simulink model "Fuel_Fault_Detection"  (R2023b)
settings: Solver=FixedStepDiscrete  StartTime=0.0  StopTime=10.0  FixedStep=0.01  RelTol=1e-3
undefined symbols (not defined in the file): sigbuilder_block
libraries: simulink x5, Median_Filter_5th_lib x2, dspsrcs4 x1
settings Model: Creator=FAbdelkarim  LastModifiedBy=Farah
settings ModelReferenceCC: EnableRefExpFcnMdlSchedulingChecks=on

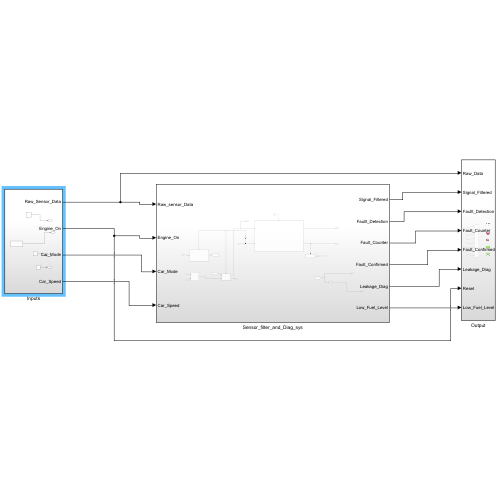
[thumbnail: Simulink's stored preview of the top-level diagram]
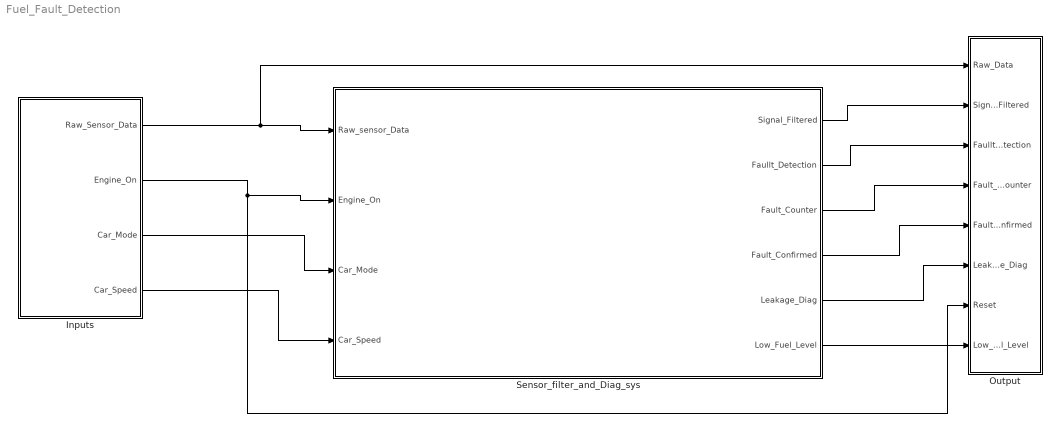
== system Fuel_Fault_Detection ==
  Inputs : Subsystem
  Output : Subsystem
  Sensor_filter_and_Diag_sys : Subsystem
  wires:
  Inputs/1(Raw_Sensor_Data) -> Output/1(Raw_Data), Sensor_filter_and_Diag_sys/1(Raw_sensor_Data)
  Inputs/2(Engine_On) -> Output/7(Reset), Sensor_filter_and_Diag_sys/2(Engine_On)
  Sensor_filter_and_Diag_sys/2(Faullt_Detection) -> Output/3(Faullt_Detection)
  Sensor_filter_and_Diag_sys/3(Fault_Counter) -> Output/4(Fault_Counter)
  Sensor_filter_and_Diag_sys/4(Fault_Confirmed) -> Output/5(Fault_Confirmed)
  Sensor_filter_and_Diag_sys/1(Signal_Filtered) -> Output/2(Signal_Filtered)
  Sensor_filter_and_Diag_sys/5(Leakage_Diag) -> Output/6(Leakage_Diag)
  Inputs/3(Car_Mode) -> Sensor_filter_and_Diag_sys/3(Car_Mode)
  Inputs/4(Car_Speed) -> Sensor_filter_and_Diag_sys/4(Car_Speed)
  Sensor_filter_and_Diag_sys/6(Low_Fuel_Level) -> Output/8(Low_Fuel_Level)

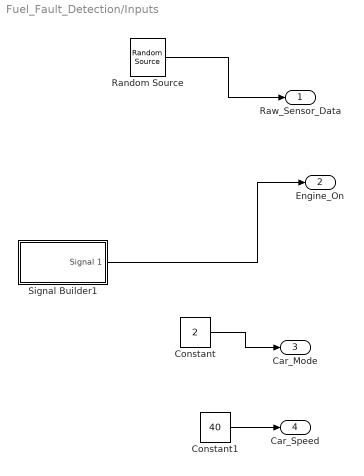
== system Fuel_Fault_Detection/Inputs ==
  Constant : Constant  Value=2
  Constant1 : Constant  Value=40
  Random Source : dspsrcs4/Random Source  SrcType=Uniform  NormMethod=Ziggurat  CltLength=12  MinVal=10  MaxVal=30  MeanVal=0  VarVal=1  RepMode=Not repeatable  rawSeed=1  IsInherit=off  SampMode=Discrete  SampTime=0.02  SampFrame=1  DataType=Double  OutComplex=Real  OutputFrames=off
  Signal Builder1 : Subsystem  Tag=STV Subsys  LoadFcn=sigbuilder_block('load');  StartFcn=sigbuilder_block('start');  StopFcn=sigbuilder_block('stop');  ClipboardFcn=sigbuilder_block('clipboard');  mask(Sigbuilder block){tuvar=[0:10]}
      mask help: Simulink:masks:SigbuilderBlock_MD
      mask init:
      | if ~strcmp(get_param(bdroot(gcbh),'SimulationStatus'),'stopped') tuvar = sigbuilder_block('maskInit'); end
      settings: CopyFcn=sigbuilder_block('copy');  DeleteFcn=sigbuilder_block('delete');  ModelCloseFcn=sigbuilder_block('modelClose');  PreSaveFcn=sigbuilder_block('preSave');  PauseFcn=sigbuilder_block('pause');  ContinueFcn=sigbuilder_block('continue');  NameChangeFcn=sigbuilder_block('namechange');  OpenFcn=sigbuilder_block('open',[437.6 199.2 550.4 400 ]);  CloseFcn=sigbuilder_block('close');
      mask Display: plot(0, 0, 100, 100,[2, 2, 32, 32, 2], [68, 8, 8, 68, 68],[32, 2], [38, 38], [32, 19, 2],[53, 60, 44], [32, 17, 17, 2],[16, 16, 31, 31]);txt = getActiveGroup(gcbh);text(2, 100, txt,'verticalAlignment', 'top');
  Raw_Sensor_Data : Outport
  Engine_On : Outport  Port=2
  Car_Mode : Outport  Port=3
  Car_Speed : Outport  Port=4
  wires:
  Random Source/1 -> Raw_Sensor_Data/1
  Signal Builder1/1(Signal 1) -> Engine_On/1
  Constant/1 -> Car_Mode/1
  Constant1/1 -> Car_Speed/1

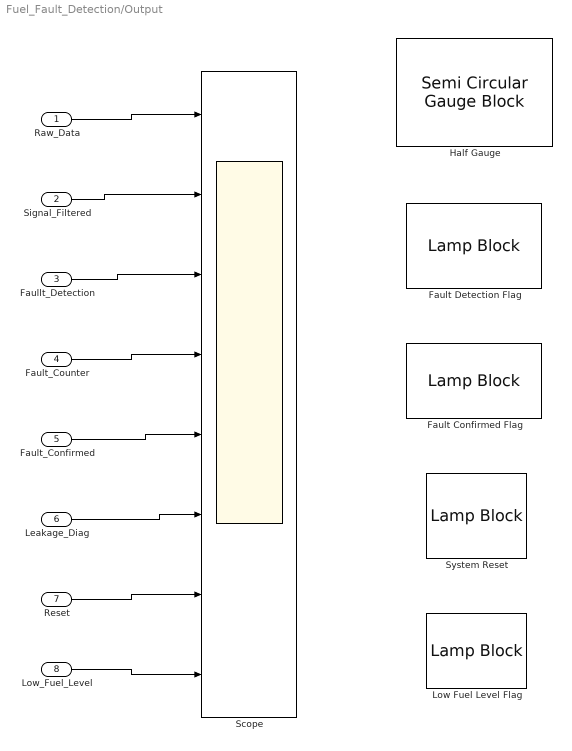
== system Fuel_Fault_Detection/Output ==
  Raw_Data : Inport
  Signal_Filtered : Inport  Port=2
  Faullt_Detection : Inport  Port=3
  Fault_Counter : Inport  Port=4
  Fault_Confirmed : Inport  Port=5
  Leakage_Diag : Inport  Port=6
  Reset : Inport  Port=7
  Low_Fuel_Level : Inport  Port=8
  Fault Confirmed Flag : LampBlock  LabelPosition=Bottom
  Fault Detection Flag : LampBlock  LabelPosition=Bottom
  Half Gauge : SemiCircularGaugeBlock
  Low Fuel Level Flag : LampBlock  LabelPosition=Bottom
  Scope : Scope  NumInputPorts=8
  System Reset : LampBlock  LabelPosition=Bottom
  wires:
  Raw_Data/1 -> Scope/1
  Signal_Filtered/1 -> Scope/2
  Faullt_Detection/1 -> Scope/3
  Fault_Counter/1 -> Scope/4
  Fault_Confirmed/1 -> Scope/5
  Leakage_Diag/1 -> Scope/6
  Reset/1 -> Scope/7
  Low_Fuel_Level/1 -> Scope/8

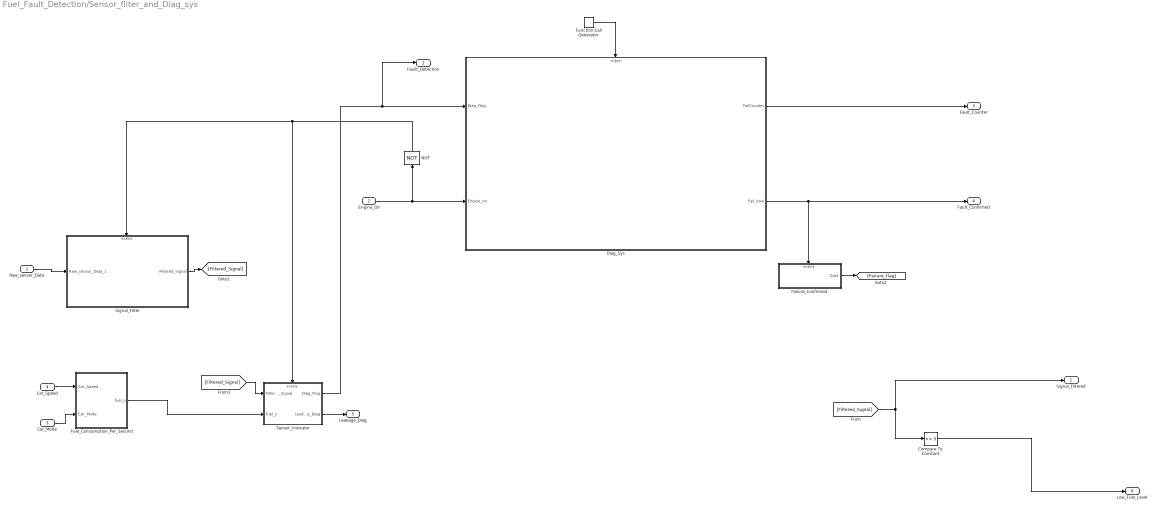
== system Fuel_Fault_Detection/Sensor_filter_and_Diag_sys ==
  Raw_sensor_Data : Inport
  Engine_On : Inport  Port=2
  Car_Mode : Inport  Port=3
  Car_Speed : Inport  Port=4
  Compare To Constant : simulink/Logic and Bit Operations/Compare To Constant  relop=<=  const=5  OutDataTypeStr=boolean
  Diag_Sys : Subsystem  TreatAsAtomicUnit=on
  Failure_Confirmed : Subsystem  TreatAsAtomicUnit=on
  Fuel_Consumption_Per_Second : Stateflow chart  TreatAsAtomicUnit=on
  Function-Call Generator : simulink/Ports & Subsystems/Function-Call Generator  sample_time=0.1  numberOfIterations=1  DisallowWideOutput=off
  NOT : Logic  Operator=NOT  IconShape=distinctive  AllPortsSameDT=off  OutDataTypeStr=boolean
  Sensor_Indicator : Subsystem  TreatAsAtomicUnit=on
  Signal_Filter : Subsystem  TreatAsAtomicUnit=on
  Signal_Filtered : Outport
  Faullt_Detection : Outport  Port=2
  Fault_Counter : Outport  Port=3
  Fault_Confirmed : Outport  Port=4
  Leakage_Diag : Outport  Port=5
  Low_Fuel_Level : Outport  Port=6
  wires:
  Raw_sensor_Data/1 -> Signal_Filter/1(Raw_sensor_Data_1)
  Diag_Sys/1(FailCounter) -> Fault_Counter/1
  Diag_Sys/2(Fail_bool) -> Fault_Confirmed/1, Failure_Confirmed/Enable
  Function-Call Generator/1 -> Diag_Sys/Trigger
  Engine_On/1 -> Diag_Sys/2(Engine_on), NOT/1
  Signal_Filter/1(Filtered_Signal) -> [Filtered_Signal]
  Failure_Confirmed/1(Out1) -> [Failure_flag]
  [Filtered_Signal] -> Signal_Filtered/1, Compare To Constant/1
  [Filtered_Signal] -> Sensor_Indicator/1(Filtered_Signal)
  Car_Speed/1 -> Fuel_Consumption_Per_Second/1(Car_Speed)
  Car_Mode/1 -> Fuel_Consumption_Per_Second/2(Car_Mode)
  Fuel_Consumption_Per_Second/1(fuel_s) -> Sensor_Indicator/2(fuel_s)
  Sensor_Indicator/1(Diag_Flag) -> Faullt_Detection/1, Diag_Sys/1(Diag_Flag)
  Sensor_Indicator/2(Leakage_Diag) -> Leakage_Diag/1
  NOT/1 -> Signal_Filter/Enable, Sensor_Indicator/Enable
  Compare To Constant/1 -> Low_Fuel_Level/1

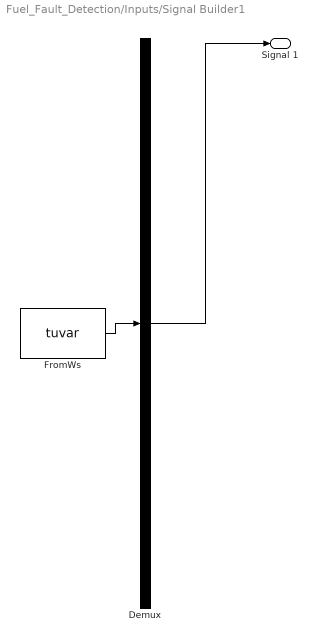
== system Fuel_Fault_Detection/Inputs/Signal Builder1 ==
  Demux : Demux  Tag=STV Demux  Outputs=1
      settings: DisplayOption=none
  FromWs : FromWorkspace  Tag=STV FromWs  VariableName=tuvar
      SigBuilderData=|
      | common.afterFinalStr = 'Extrapolate'
      | common.sampleTime = 0
      | dataSet.timeRange = [0 10]
      | dataSet.name = 'Group 1'
      | sbobj.Groups.Name = 'Group 1'
      | sbobj.Groups.Signals.Name = 'Signal 1'
      | sbobj.Groups.Signals.XData = [0 2.02 2.02 2.4 2.4 10]
      | sbobj.Groups.Signals.YData = [0 0 1 1 0 0]
  Signal 1 : Outport  Tag=STV Outport
  wires:
  Demux/1 -> Signal 1/1
  FromWs/1 -> Demux/1

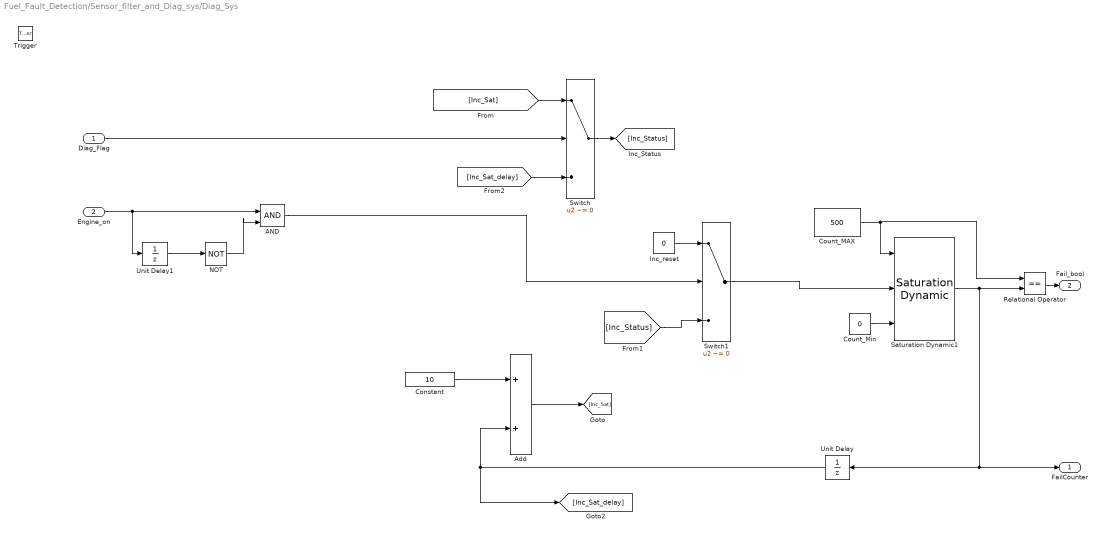
== system Fuel_Fault_Detection/Sensor_filter_and_Diag_sys/Diag_Sys ==
  Diag_Flag : Inport
  Engine_on : Inport  Port=2
  Trigger : TriggerPort  TriggerType=function-call  VariantControl=(inherit)  PortDimensions=1
  AND : Logic  IconShape=distinctive  AllPortsSameDT=off  OutDataTypeStr=boolean
  Add : Sum
  Constant : Constant  Value=10
  Count_MAX : Constant  Value=500
  Count_Min : Constant  Value=0
  Inc_reset : Constant  Value=0
  NOT : Logic  Operator=NOT  IconShape=distinctive  AllPortsSameDT=off  OutDataTypeStr=boolean
  Relational Operator : RelationalOperator  Operator===  OutDataTypeStr=boolean  RndMeth=Simplest  InputSameDT=off
  Saturation Dynamic1 : simulink/Discontinuities/Saturation Dynamic  OutMin=[]  OutMax=[]  OutDataTypeStr=Inherit: Same as second input  OutDataType=fixdt(1, 16)  OutScaling=2^-10  DoSatur=off
  Switch : Switch  Criteria=u2 ~= 0  SaturateOnIntegerOverflow=off  InputSameDT=off
  Switch1 : Switch  Criteria=u2 ~= 0  SaturateOnIntegerOverflow=off  InputSameDT=off
  Unit Delay : UnitDelay  SampleTime=-1  HasFrameUpgradeWarning=on
  Unit Delay1 : UnitDelay  SampleTime=-1  HasFrameUpgradeWarning=on
  FailCounter : Outport
  Fail_bool : Outport  Port=2
  wires:
  Switch/1 -> [Inc_Status]
  Relational Operator/1 -> Fail_bool/1
  Saturation Dynamic1/1 -> FailCounter/1, Unit Delay/1, Relational Operator/2
  Unit Delay1/1 -> NOT/1
  [Inc_Status] -> Switch1/3
  Inc_reset/1 -> Switch1/1
  Engine_on/1 -> AND/1, Unit Delay1/1
  Count_Min/1 -> Saturation Dynamic1/3
  NOT/1 -> AND/2
  [Inc_Sat_delay] -> Switch/3
  Switch1/1 -> Saturation Dynamic1/2
  AND/1 -> Switch1/2
  Unit Delay/1 -> [Inc_Sat_delay], Add/2
  [Inc_Sat] -> Switch/1
  Constant/1 -> Add/1
  Diag_Flag/1 -> Switch/2
  Count_MAX/1 -> Saturation Dynamic1/1, Relational Operator/1
  Add/1 -> [Inc_Sat]

== system Fuel_Fault_Detection/Sensor_filter_and_Diag_sys/Failure_Confirmed ==
  Enable : EnablePort
  Constant : Constant  Value=-1
  Out1 : Outport
  wires:
  Constant/1 -> Out1/1

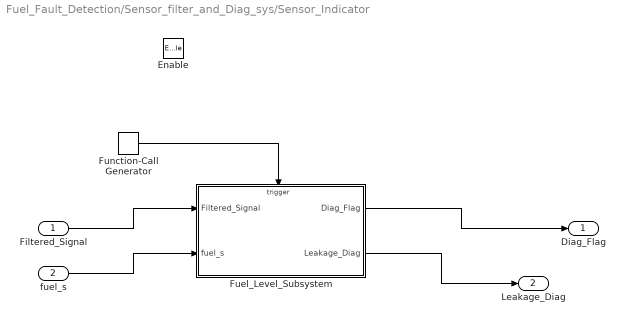
== system Fuel_Fault_Detection/Sensor_filter_and_Diag_sys/Sensor_Indicator ==
  Filtered_Signal : Inport
  fuel_s : Inport  Port=2
  Enable : EnablePort
  Fuel_Level_Subsystem : Subsystem  TreatAsAtomicUnit=on
  Function-Call Generator : simulink/Ports & Subsystems/Function-Call Generator  sample_time=1  numberOfIterations=1  DisallowWideOutput=off
  Diag_Flag : Outport
  Leakage_Diag : Outport  Port=2
  wires:
  Filtered_Signal/1 -> Fuel_Level_Subsystem/1(Filtered_Signal)
  Fuel_Level_Subsystem/1(Diag_Flag) -> Diag_Flag/1
  Function-Call Generator/1 -> Fuel_Level_Subsystem/Trigger
  fuel_s/1 -> Fuel_Level_Subsystem/2(fuel_s)
  Fuel_Level_Subsystem/2(Leakage_Diag) -> Leakage_Diag/1

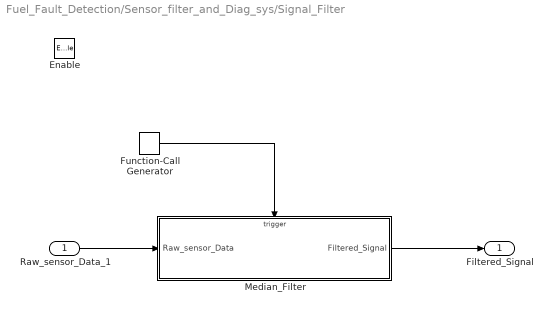
== system Fuel_Fault_Detection/Sensor_filter_and_Diag_sys/Signal_Filter ==
  Raw_sensor_Data_1 : Inport
  Enable : EnablePort
  Function-Call Generator : simulink/Ports & Subsystems/Function-Call Generator  sample_time=0.02  numberOfIterations=1  DisallowWideOutput=off
  Median_Filter : Subsystem
  Filtered_Signal : Outport
  wires:
  Raw_sensor_Data_1/1 -> Median_Filter/1(Raw_sensor_Data)
  Median_Filter/1(Filtered_Signal) -> Filtered_Signal/1
  Function-Call Generator/1 -> Median_Filter/Trigger

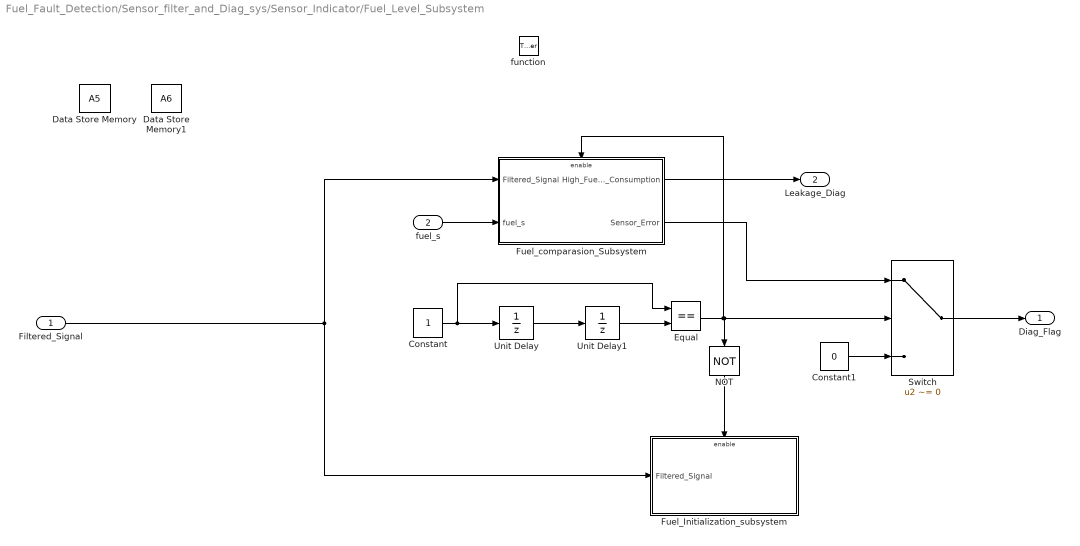
== system Fuel_Fault_Detection/Sensor_filter_and_Diag_sys/Sensor_Indicator/Fuel_Level_Subsystem ==
  Filtered_Signal : Inport
  fuel_s : Inport  Port=2
  function : TriggerPort  TriggerType=function-call  VariantControl=(inherit)
  Constant : Constant  SampleTime=-1
  Constant1 : Constant  Value=0
  Data Store Memory : DataStoreMemory  DataStoreName=A5  WriteAfterWriteMsg=warning  ShowAdditionalParam=off
  Data Store Memory1 : DataStoreMemory  DataStoreName=A6  WriteAfterWriteMsg=warning  ShowAdditionalParam=off
  Equal : RelationalOperator  Operator===  OutDataTypeStr=boolean  RndMeth=Simplest  InputSameDT=off
  Fuel_Initialization_subsystem : Subsystem  TreatAsAtomicUnit=on
  Fuel_comparasion_Subsystem : Subsystem  TreatAsAtomicUnit=on
  NOT : Logic  Operator=NOT  IconShape=distinctive  AllPortsSameDT=off  OutDataTypeStr=boolean
  Switch : Switch  Criteria=u2 ~= 0  SaturateOnIntegerOverflow=off  InputSameDT=off
  Unit Delay : UnitDelay  SampleTime=-1  HasFrameUpgradeWarning=on
  Unit Delay1 : UnitDelay  SampleTime=-1  HasFrameUpgradeWarning=on
  Diag_Flag : Outport
  Leakage_Diag : Outport  Port=2
  wires:
  Unit Delay1/1 -> Equal/2
  Equal/1 -> Fuel_comparasion_Subsystem/Enable, Switch/2, NOT/1
  Unit Delay/1 -> Unit Delay1/1
  Filtered_Signal/1 -> Fuel_Initialization_subsystem/1(Filtered_Signal), Fuel_comparasion_Subsystem/1(Filtered_Signal)
  Switch/1 -> Diag_Flag/1
  Constant/1 -> Equal/1, Unit Delay/1
  NOT/1 -> Fuel_Initialization_subsystem/Enable
  Fuel_comparasion_Subsystem/2(Sensor_Error) -> Switch/1
  fuel_s/1 -> Fuel_comparasion_Subsystem/2(fuel_s)
  Fuel_comparasion_Subsystem/1(High_Fuel_Consumption) -> Leakage_Diag/1
  Constant1/1 -> Switch/3

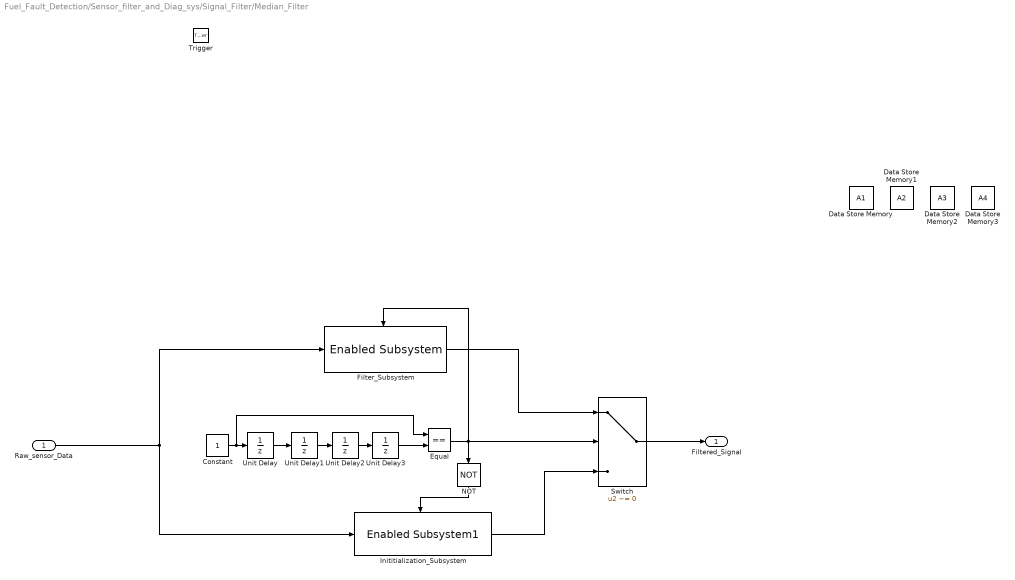
== system Fuel_Fault_Detection/Sensor_filter_and_Diag_sys/Signal_Filter/Median_Filter ==
  Raw_sensor_Data : Inport
  Trigger : TriggerPort  TriggerType=function-call  VariantControl=(inherit)  PortDimensions=1
  Constant : Constant  SampleTime=-1
  Data Store Memory : DataStoreMemory  DataStoreName=A1  WriteAfterWriteMsg=warning  ShowAdditionalParam=off
  Data Store Memory1 : DataStoreMemory  DataStoreName=A2  WriteAfterWriteMsg=warning  ShowAdditionalParam=off
  Data Store Memory2 : DataStoreMemory  DataStoreName=A3  WriteAfterWriteMsg=warning  ShowAdditionalParam=off
  Data Store Memory3 : DataStoreMemory  DataStoreName=A4  WriteAfterWriteMsg=warning  ShowAdditionalParam=off
  Equal : RelationalOperator  Operator===  OutDataTypeStr=boolean  RndMeth=Simplest  InputSameDT=off
  Filter_Subsystem : Median_Filter_5th_lib/Median_Filter_5th/Enabled Subsystem  SystemSampleTime=-1  VariantActivationTime=update diagram  AllowFlexibleInterface=on  Latency=0  AutoFrameSizeCalculation=off
  Inititialization_Subsystem : Median_Filter_5th_lib/Median_Filter_5th/Enabled Subsystem1  SystemSampleTime=-1  VariantActivationTime=update diagram  AllowFlexibleInterface=on  Latency=0  AutoFrameSizeCalculation=off
  NOT : Logic  Operator=NOT  IconShape=distinctive  AllPortsSameDT=off  OutDataTypeStr=boolean
  Switch : Switch  Criteria=u2 ~= 0  SaturateOnIntegerOverflow=off  InputSameDT=off
  Unit Delay{,1..3} (4 alike) : UnitDelay  SampleTime=-1  HasFrameUpgradeWarning=on
  Filtered_Signal : Outport
  wires:
  Unit Delay1/1 -> Unit Delay2/1
  Filter_Subsystem/1 -> Switch/1
  Constant/1 -> Equal/1, Unit Delay/1
  Raw_sensor_Data/1 -> Filter_Subsystem/1, Inititialization_Subsystem/1
  Equal/1 -> Switch/2, NOT/1, Filter_Subsystem/Enable
  Switch/1 -> Filtered_Signal/1
  Unit Delay/1 -> Unit Delay1/1
  NOT/1 -> Inititialization_Subsystem/Enable
  Inititialization_Subsystem/1 -> Switch/3
  Unit Delay2/1 -> Unit Delay3/1
  Unit Delay3/1 -> Equal/2

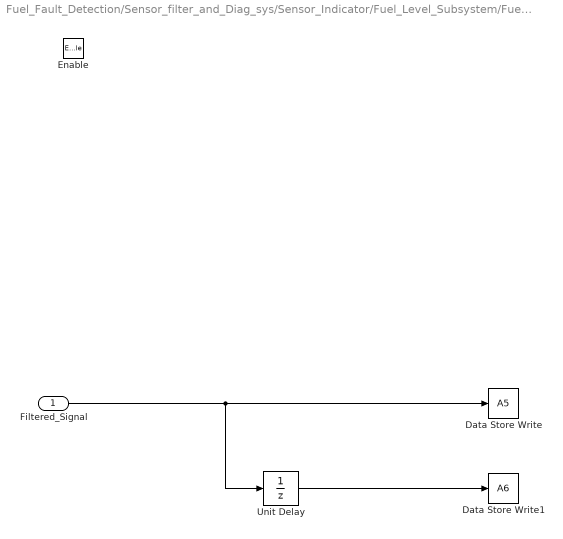
== system Fuel_Fault_Detection/Sensor_filter_and_Diag_sys/Sensor_Indicator/Fuel_Level_Subsystem/Fuel_Initialization_subsystem ==
  Filtered_Signal : Inport
  Enable : EnablePort
  Data Store Write : DataStoreWrite  DataStoreName=A5  IndexOptions=Index vector (dialog)  Indices=1  OutputSizes=1
  Data Store Write1 : DataStoreWrite  DataStoreName=A6  IndexOptions=Index vector (dialog)  Indices=1  OutputSizes=1
  Unit Delay : UnitDelay  SampleTime=-1  HasFrameUpgradeWarning=on
  wires:
  Filtered_Signal/1 -> Data Store Write/1, Unit Delay/1
  Unit Delay/1 -> Data Store Write1/1

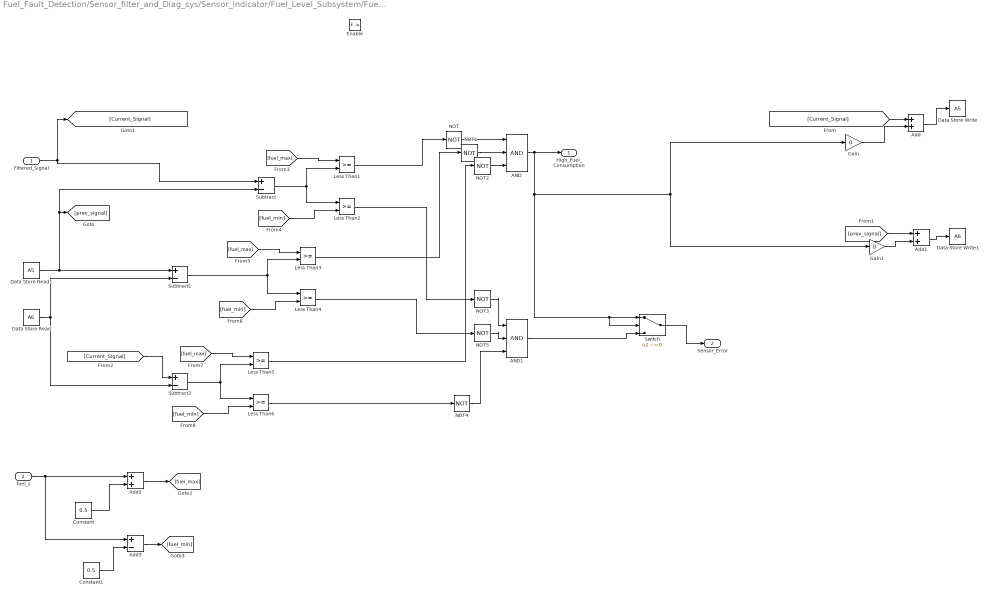
== system Fuel_Fault_Detection/Sensor_filter_and_Diag_sys/Sensor_Indicator/Fuel_Level_Subsystem/Fuel_comparasion_Subsystem ==
  Filtered_Signal : Inport
  fuel_s : Inport  Port=2
  Enable : EnablePort
  AND : Logic  Inputs=3  IconShape=distinctive  AllPortsSameDT=off  OutDataTypeStr=boolean
  AND1 : Logic  Inputs=3  IconShape=distinctive  AllPortsSameDT=off  OutDataTypeStr=boolean
  Add : Sum
  Add1 : Sum
  Add2 : Sum
  Add3 : Sum  Inputs=+-
  Constant : Constant  Value=0.5
  Constant1 : Constant  Value=0.5
  Data Store Read : DataStoreRead  DataStoreName=A6  IndexOptions=Index vector (dialog)  Indices=1  OutputSizes=1
  Data Store Read1 : DataStoreRead  DataStoreName=A5  IndexOptions=Index vector (dialog)  Indices=1  OutputSizes=1
  Data Store Write : DataStoreWrite  DataStoreName=A5  IndexOptions=Index vector (dialog)  Indices=1  OutputSizes=1
  Data Store Write1 : DataStoreWrite  DataStoreName=A6  IndexOptions=Index vector (dialog)  Indices=1  OutputSizes=1
  Gain : Gain  Gain=0
  Gain1 : Gain  Gain=0
  Less Than{1..6} (6 alike) : RelationalOperator  OutDataTypeStr=boolean  RndMeth=Simplest  InputSameDT=off
  NOT{,1..5} (6 alike) : Logic  Operator=NOT  IconShape=distinctive  AllPortsSameDT=off  OutDataTypeStr=boolean
  Subtract : Sum  Inputs=+-
  Subtract1 : Sum  Inputs=+-
  Subtract2 : Sum  Inputs=+-
  Switch : Switch  Criteria=u2 ~= 0  SaturateOnIntegerOverflow=off  InputSameDT=off
  High_Fuel_Consumption : Outport
  Sensor_Error : Outport  Port=2
  wires:
  AND/1 -> High_Fuel_Consumption/1, Switch/2, Switch/1, Gain1/1, Gain/1
  Gain/1 -> Add/2
  Gain1/1 -> Add1/2
  Add/1 -> Data Store Write/1
  Add1/1 -> Data Store Write1/1
  Data Store Read1/1 -> Subtract/2, [prev_signal], Subtract1/1
  Filtered_Signal/1 -> [Current_Signal], Subtract/1
  [Current_Signal] -> Add/1
  [prev_signal] -> Add1/1
  Data Store Read/1 -> Subtract1/2, Subtract2/2
  Constant/1 -> Add2/2
  fuel_s/1 -> Add3/1, Add2/1
  Constant1/1 -> Add3/2
  [Current_Signal] -> Subtract2/1
  Add2/1 -> [fuel_max]
  Add3/1 -> [fuel_min]
  Subtract/1 -> Less Than1/2, Less Than2/1
  [fuel_max] -> Less Than1/1
  [fuel_min] -> Less Than2/2
  [fuel_min] -> Less Than4/2
  Subtract1/1 -> Less Than4/1, Less Than3/2
  [fuel_max] -> Less Than3/1
  [fuel_min] -> Less Than6/2
  Subtract2/1 -> Less Than5/2, Less Than6/1
  [fuel_max] -> Less Than5/1
  Less Than1/1 -> NOT/1
  Less Than3/1 -> NOT1/1
  Less Than5/1 -> NOT2/1
  NOT/1 -> AND/1
  NOT1/1 -> AND/2
  NOT2/1 -> AND/3
  Less Than2/1 -> NOT3/1
  Less Than4/1 -> NOT5/1
  Less Than6/1 -> NOT4/1
  NOT3/1 -> AND1/1
  NOT5/1 -> AND1/2
  NOT4/1 -> AND1/3
  AND1/1 -> Switch/3
  Switch/1 -> Sensor_Error/1

== stateflow chart Fuel_Fault_Detection/Sensor_filter_and_Diag_sys/Fuel_Consumption_Per_Second ==
  state Parking_Neutral_Mode
    entry:
    fuel_s=0.5;
  state Driving_Mode
    state D_Low_speed
      entry:
      fuel_s=1;
    state D_Mid_Speed
      entry:
      fuel_s=3;
    state D_Very_High_Speed
      entry:
      fuel_s=6;
    state D_high_Speed
      entry:
      fuel_s=5;
    (default) -> D_Low_speed
    D_Low_speed -> D_Mid_Speed : [Car_Speed>=30]
    D_Mid_Speed -> D_Low_speed [order 1] : [Car_Speed<30]
    D_Mid_Speed -> D_high_Speed [order 2] : [Car_Speed>=70&& Car_Speed<100]
    D_high_Speed -> D_Mid_Speed [order 1] : [Car_Speed<70]
    D_high_Speed -> D_Very_High_Speed [order 2] : [Car_Speed>=100]
    D_Very_High_Speed -> D_high_Speed : [Car_Speed<100]
  state Reverse_Mode
    state Reverse_Low_speed
      entry:
      fuel_s=2;
    state Reverse_High_Speed
      entry:
      fuel_s=4;
    (default) -> Reverse_Low_speed
    Reverse_Low_speed -> Reverse_High_Speed : [Car_Speed>=20]
    Reverse_High_Speed -> Reverse_Low_speed : [Car_Speed<20]
  (default) -> Parking_Neutral_Mode
  Parking_Neutral_Mode -> Driving_Mode [order 2] : [Car_Mode==2]
  Driving_Mode -> Parking_Neutral_Mode [order 1] : [Car_Mode==0]
  Parking_Neutral_Mode -> Reverse_Mode [order 1] : [Car_Mode==1]
  Reverse_Mode -> Parking_Neutral_Mode [order 1] : [Car_Mode==0]
  Reverse_Mode -> Driving_Mode [order 2] : [Car_Mode==2]
  Driving_Mode -> Reverse_Mode [order 2] : [Car_Mode==1]
  data: Car_Speed input; Car_Mode input; fuel_s output
